simulink model "simulation_plaque"  (R2019a)
settings: Solver=ode45  StartTime=0.0  StopTime=tfin  FixedStep=0.001  RelTol=1e-09  EnableMultiTasking=on
undefined symbols (not defined in the file or in its folder): Ae, As, Be, g, Jx, LL, mP, mS, phi_1, RR, Vmax, XA, XB, XC, XD, XE, XF, YA, YB, YC, YD, YE, YF, z_re
settings Model: Creator=delafontaine  LastModifiedBy=arsp2701
settings SolverCC: AlgebraicLoopSolver=LineSearch
settings DataIOCC: LimitDataPoints=on  SaveFormat=Array  SignalLoggingSaveFormat=ModelDataLogs  ReturnWorkspaceOutputs=off
settings OptimizationCC: LifeSpan=inf
settings DebuggingCC: UnderspecifiedInitializationDetection=Classic  MergeDetectMultiDrivingBlocksExec=none  MultiTaskDSMMsg=warning  MultiTaskCondExecSysMsg=none  SFUnexpectedBacktrackingDiag=warning  SFNoUnconditionalDefaultTransitionDiag=warning  SFExecutionAtInitializationDiag=none  UnderSpecifiedDimensionMsg=warning  ArithmeticOperatorsInVariantConditions=warning
settings HardwareCC: ProdBitPerPointer=32  ProdBitPerSizeT=32  ProdBitPerPtrDiffT=32  ProdLargestAtomicFloat=None  ProdIntDivRoundTo=Undefined  ProdEndianess=Unspecified  ProdWordSize=32  ProdHWDeviceType=32-bit Generic
settings ModelReferenceCC: PropagateSignalLabelsOutOfModel=off
settings SFSimCC: SimUseLocalCustomCode=off
settings RTWCC: RTWUseLocalCustomCode=off
settings CodeAppCC: StateflowObjectComments=on
settings GRTTargetCC: TargetLangStandard=C89/C90 (ANSI)  GeneratePreprocessorConditionals=Disable all
settings ConfigComp: CovMetricSettings=dw  CovHtmlReporting=on  CovSaveCumulativeToWorkspaceVar=on  CovSaveSingleToWorkspaceVar=on  CovExternalEMLEnable=off  CovSFcnEnable=off

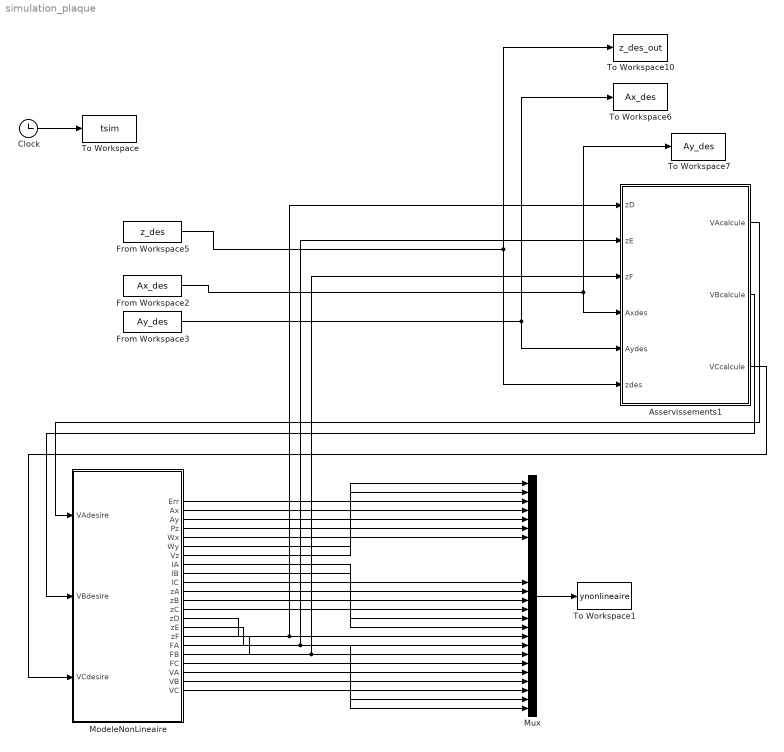
== system simulation_plaque ==
  Asservissements1 : Subsystem
      mask help: Simulink:masks:GenSFuncDesc_MD
      mask Help: eval('feval(''rtwprivate'',''rtwhelpview'',''rtw_sfcn_block'')');
  Clock : Clock
  From Workspace2 : FromWorkspace  VariableName=Ax_des  SampleTime=0  Interpolate=off  OutputAfterFinalValue=Holding final value
  From Workspace3 : FromWorkspace  VariableName=Ay_des  SampleTime=0  Interpolate=off  OutputAfterFinalValue=Holding final value
  From Workspace5 : FromWorkspace  VariableName=z_des  SampleTime=0  Interpolate=off  OutputAfterFinalValue=Holding final value
  ModeleNonLineaire : Subsystem
      mask help: Simulink:masks:GenSFuncDesc_MD
      mask Help: eval('feval(''rtwprivate'',''rtwhelpview'',''rtw_sfcn_block'')');
  Mux : Mux  Inputs=26
  To Workspace : ToWorkspace  VariableName=tsim  SampleTime=-1
  To Workspace1 : ToWorkspace  VariableName=ynonlineaire  SampleTime=-1
  To Workspace10 : ToWorkspace  VariableName=z_des_out  SampleTime=-1
  To Workspace6 : ToWorkspace  VariableName=Ax_des  SampleTime=-1
  To Workspace7 : ToWorkspace  VariableName=Ay_des  SampleTime=-1
  wires:
  Mux/1 -> To Workspace1/1
  Clock/1 -> To Workspace/1
  From Workspace5/1 -> Asservissements1/6(zdes), To Workspace10/1
  ModeleNonLineaire/2(Ax) -> Mux/2
  ModeleNonLineaire/3(Ay) -> Mux/3
  ModeleNonLineaire/4(Pz) -> Mux/4
  ModeleNonLineaire/5(Wx) -> Mux/5
  ModeleNonLineaire/6(Wy) -> Mux/6
  ModeleNonLineaire/7(Vz) -> Mux/7
  ModeleNonLineaire/8(IA) -> Mux/12
  ModeleNonLineaire/9(IB) -> Mux/13
  ModeleNonLineaire/10(IC) -> Mux/14
  From Workspace3/1 -> To Workspace6/1, Asservissements1/5(Aydes)
  From Workspace2/1 -> To Workspace7/1, Asservissements1/4(Axdes)
  ModeleNonLineaire/17(FA) -> Mux/21
  ModeleNonLineaire/18(FB) -> Mux/22
  ModeleNonLineaire/19(FC) -> Mux/23
  ModeleNonLineaire/20(VA) -> Mux/24
  ModeleNonLineaire/21(VB) -> Mux/25
  ModeleNonLineaire/22(VC) -> Mux/26
  ModeleNonLineaire/14(zD) -> Asservissements1/1(zD), Mux/18
  ModeleNonLineaire/15(zE) -> Asservissements1/2(zE), Mux/19
  ModeleNonLineaire/16(zF) -> Asservissements1/3(zF), Mux/20
  ModeleNonLineaire/11(zA) -> Mux/15
  ModeleNonLineaire/12(zB) -> Mux/16
  ModeleNonLineaire/13(zC) -> Mux/17
  Asservissements1/1(VAcalcule) -> ModeleNonLineaire/1(VAdesire)
  Asservissements1/2(VBcalcule) -> ModeleNonLineaire/2(VBdesire)
  Asservissements1/3(VCcalcule) -> ModeleNonLineaire/3(VCdesire)
  ModeleNonLineaire/1("Err ") -> Mux/1

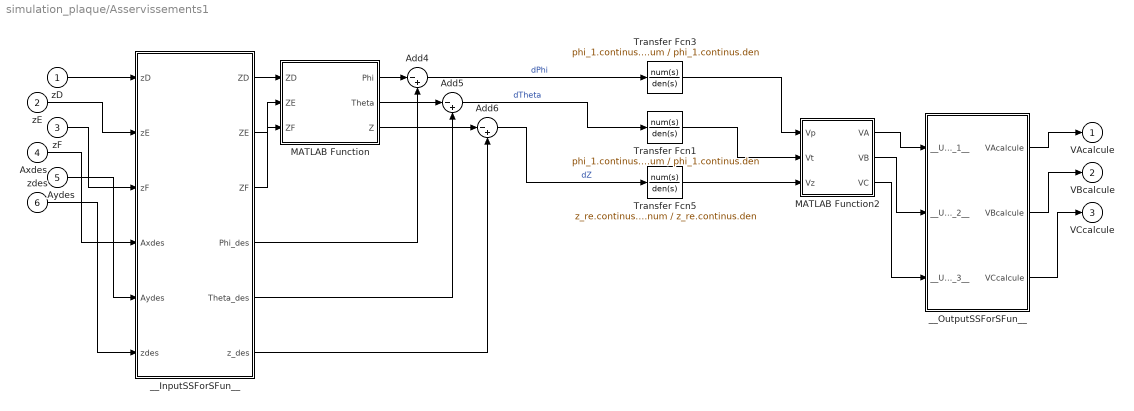
== system simulation_plaque/Asservissements1 ==
  zD : Inport
  zE : Inport  Port=2
  zF : Inport  Port=3
  Axdes : Inport  Port=4
  Aydes : Inport  Port=5
  zdes : Inport  Port=6
  Add4 : Sum  Inputs=|-+
  Add5 : Sum  Inputs=|-+
  Add6 : Sum  Inputs=|-+
  MATLAB Function : MATLAB Function  TreatAsAtomicUnit=on
  MATLAB Function2 : MATLAB Function  TreatAsAtomicUnit=on
  Transfer Fcn1 : TransferFcn  Numerator=phi_1.continus.num  Denominator=phi_1.continus.den
  Transfer Fcn3 : TransferFcn  Numerator=phi_1.continus.num  Denominator=phi_1.continus.den
  Transfer Fcn5 : TransferFcn  Numerator=z_re.continus.num  Denominator=z_re.continus.den
  __InputSSForSFun__ : Subsystem
  __OutputSSForSFun__ : Subsystem
  VAcalcule : Outport
  VBcalcule : Outport  Port=2
  VCcalcule : Outport  Port=3
  wires:
  zD/1 -> __InputSSForSFun__/1(zD)
  zE/1 -> __InputSSForSFun__/2(zE)
  zF/1 -> __InputSSForSFun__/3(zF)
  Axdes/1 -> __InputSSForSFun__/4(Axdes)
  Aydes/1 -> __InputSSForSFun__/5(Aydes)
  zdes/1 -> __InputSSForSFun__/6(zdes)
  __InputSSForSFun__/1(ZD) -> MATLAB Function/1(ZD)
  __OutputSSForSFun__/1(VAcalcule) -> VAcalcule/1
  __OutputSSForSFun__/2(VBcalcule) -> VBcalcule/1
  __OutputSSForSFun__/3(VCcalcule) -> VCcalcule/1
  MATLAB Function/1(Phi) -> Add4/1
  MATLAB Function/3(Z) -> Add6/1
  MATLAB Function2/1(VA) -> __OutputSSForSFun__/1(__UniqueInportName__1__)
  MATLAB Function2/2(VB) -> __OutputSSForSFun__/2(__UniqueInportName__2__)
  MATLAB Function2/3(VC) -> __OutputSSForSFun__/3(__UniqueInportName__3__)
  MATLAB Function/2(Theta) -> Add5/1
  Add4/1 -> Transfer Fcn3/1  "dPhi"
  Transfer Fcn3/1 -> MATLAB Function2/1(Vp)
  Transfer Fcn1/1 -> MATLAB Function2/2(Vt)
  Add5/1 -> Transfer Fcn1/1  "dTheta"
  Transfer Fcn5/1 -> MATLAB Function2/3(Vz)
  Add6/1 -> Transfer Fcn5/1  "dZ"
  __InputSSForSFun__/2(ZE) -> MATLAB Function/2(ZE)
  __InputSSForSFun__/3(ZF) -> MATLAB Function/3(ZF)
  __InputSSForSFun__/4(Phi_des) -> Add4/2
  __InputSSForSFun__/5(Theta_des) -> Add5/2
  __InputSSForSFun__/6(z_des) -> Add6/2

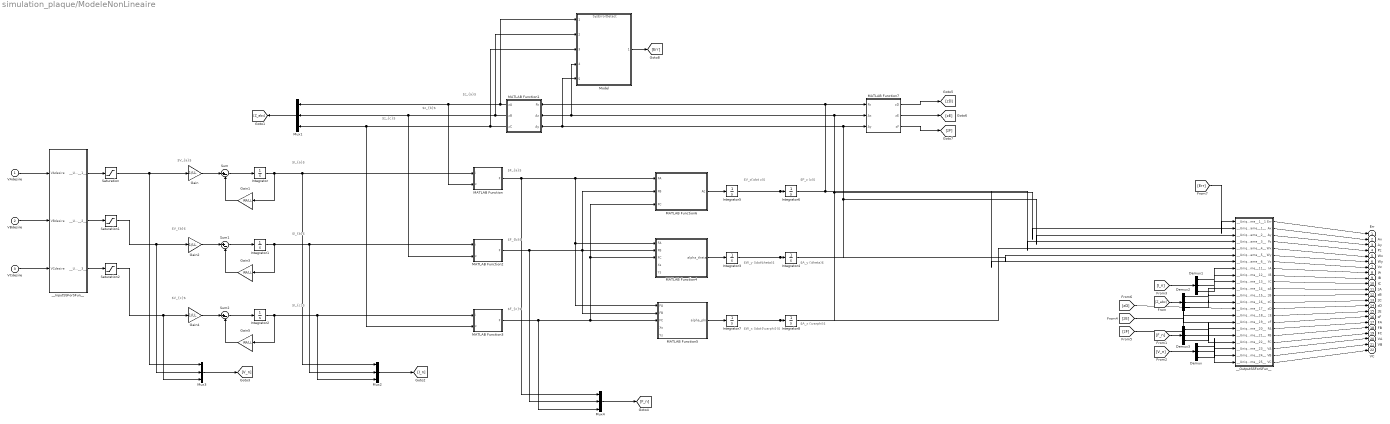
== system simulation_plaque/ModeleNonLineaire ==
  note: $z_{c}$
  note: $I_{a}$
  note: $I_{c}$
  note: $z_{b}$
  note: $F_{a}$
  note: $V_{b}$
  note: $F_{b}$
  note: $F_{c}$
  note: $V_{c}$
  note: $V_z(\dot z)$
  note: $z_{a}$
  note: $I_{b}$
  note: $V_{a}$
  note: $A_y (\theta)$
  note: $A_x (\varphi)$
  note: $W_x (\dot{\varphi})$
  note: $W_y (\dot\theta)$
  note: $P_z (z)$
  VAdesire : Inport
  VBdesire : Inport  Port=2
  VCdesire : Inport  Port=3
  Demux{,1..3} (4 alike) : Demux  Outputs=3
  Gain : Gain  Gain=1/LL
  Gain1 : Gain  Gain=RR/LL
  Gain2 : Gain  Gain=1/LL
  Gain3 : Gain  Gain=RR/LL
  Gain4 : Gain  Gain=1/LL
  Gain5 : Gain  Gain=RR/LL
  Integrator : Integrator  InitialCondition=-0.4961
  Integrator1 : Integrator  InitialCondition=-0.4961
  Integrator2 : Integrator  InitialCondition=-0.4961
  Integrator{3..5,7..8} (5 alike) : Integrator
  Integrator6 : Integrator  InitialCondition=0.015
  MATLAB Function : MATLAB Function  TreatAsAtomicUnit=on
  MATLAB Function1 : MATLAB Function  TreatAsAtomicUnit=on
  MATLAB Function2 : MATLAB Function  TreatAsAtomicUnit=on
  MATLAB Function3 : MATLAB Function  TreatAsAtomicUnit=on
  MATLAB Function4 : MATLAB Function  TreatAsAtomicUnit=on
  MATLAB Function5 : MATLAB Function  TreatAsAtomicUnit=on
  MATLAB Function6 : MATLAB Function  TreatAsAtomicUnit=on
  MATLAB Function7 : MATLAB Function  TreatAsAtomicUnit=on
  Model : ModelReference  ModelNameDialog=SysErrorDetect.slx  SimulationMode=Normal  ModelReferenceVersion=1.36
  Mux{1..4} (4 alike) : Mux  Inputs=3
  Saturation : Saturate  UpperLimit=Vmax  LowerLimit=-Vmax
  Saturation1 : Saturate  UpperLimit=Vmax  LowerLimit=-Vmax
  Saturation2 : Saturate  UpperLimit=Vmax  LowerLimit=-Vmax
  Sum : Sum  Inputs=|+-
  Sum1 : Sum  Inputs=|+-
  Sum2 : Sum  Inputs=|+-
  __InputSSForSFun__ : Subsystem
  __OutputSSForSFun__ : Subsystem
  "Err " : Outport
  Ax : Outport  Port=2
  Ay : Outport  Port=3
  Pz : Outport  Port=4
  Wx : Outport  Port=5
  Wy : Outport  Port=6
  Vz : Outport  Port=7
  IA : Outport  Port=8
  IB : Outport  Port=9
  IC : Outport  Port=10
  zA : Outport  Port=11
  zB : Outport  Port=12
  zC : Outport  Port=13
  zD : Outport  Port=14
  zE : Outport  Port=15
  zF : Outport  Port=16
  FA : Outport  Port=17
  FB : Outport  Port=18
  FC : Outport  Port=19
  VA : Outport  Port=20
  VB : Outport  Port=21
  VC : Outport  Port=22
  wires:
  VAdesire/1 -> __InputSSForSFun__/1(VAdesire)
  VBdesire/1 -> __InputSSForSFun__/2(VBdesire)
  VCdesire/1 -> __InputSSForSFun__/3(VCdesire)
  __InputSSForSFun__/1(__UniqueOutportName__1__) -> Saturation/1
  __InputSSForSFun__/2(__UniqueOutportName__2__) -> Saturation1/1
  __InputSSForSFun__/3(__UniqueOutportName__3__) -> Saturation2/1
  __OutputSSForSFun__/2(Ax) -> Ax/1
  __OutputSSForSFun__/3(Ay) -> Ay/1
  __OutputSSForSFun__/4(Pz) -> Pz/1
  __OutputSSForSFun__/5(Wx) -> Wx/1
  __OutputSSForSFun__/6(Wy) -> Wy/1
  __OutputSSForSFun__/7(Vz) -> Vz/1
  __OutputSSForSFun__/8(IA) -> IA/1
  __OutputSSForSFun__/9(IB) -> IB/1
  __OutputSSForSFun__/10(IC) -> IC/1
  __OutputSSForSFun__/11(zA) -> zA/1
  __OutputSSForSFun__/12(zB) -> zB/1
  __OutputSSForSFun__/13(zC) -> zC/1
  __OutputSSForSFun__/14(zD) -> zD/1
  __OutputSSForSFun__/15(zE) -> zE/1
  __OutputSSForSFun__/16(zF) -> zF/1
  __OutputSSForSFun__/17(FA) -> FA/1
  __OutputSSForSFun__/18(FB) -> FB/1
  __OutputSSForSFun__/19(FC) -> FC/1
  __OutputSSForSFun__/20(VA) -> VA/1
  __OutputSSForSFun__/21(VB) -> VB/1
  __OutputSSForSFun__/22(VC) -> VC/1
  Sum2/1 -> Integrator2/1
  Integrator/1 -> MATLAB Function/1(i), Mux2/1, Gain1/1
  Integrator8/1 -> __OutputSSForSFun__/2(__UniqueInportName__1__), Model/4, MATLAB Function1/2(Ax), MATLAB Function7/2(Ax)
  Integrator1/1 -> MATLAB Function2/1(i), Mux2/2, Gain3/1
  MATLAB Function1/3(zC) -> Model/3, MATLAB Function3/2(z), Mux1/3
  MATLAB Function/1(F) -> Mux4/1, MATLAB Function6/1(FA), MATLAB Function4/1(FA), MATLAB Function5/1(FA)
  Sum1/1 -> Integrator1/1
  MATLAB Function5/1(alpha_phi) -> Integrator7/1
  MATLAB Function6/1(Az) -> Integrator5/1
  Sum/1 -> Integrator/1
  Gain3/1 -> Sum1/2
  Integrator2/1 -> Gain5/1, MATLAB Function3/1(i), Mux2/3
  Integrator7/1 -> Integrator8/1, __OutputSSForSFun__/5(__UniqueInportName__4__)
  Gain5/1 -> Sum2/2
  MATLAB Function1/1(zA) -> Model/1, MATLAB Function/2(z), Mux1/1
  Integrator6/1 -> MATLAB Function1/1(Pz), MATLAB Function7/1(Pz), __OutputSSForSFun__/4(__UniqueInportName__3__)
  Integrator3/1 -> __OutputSSForSFun__/6(__UniqueInportName__5__), Integrator4/1
  Gain2/1 -> Sum1/1
  Integrator4/1 -> Model/5, MATLAB Function1/3(Ay), MATLAB Function7/3(Ay), __OutputSSForSFun__/3(__UniqueInportName__2__)
  MATLAB Function4/1(alpha_theta) -> Integrator3/1
  MATLAB Function3/1(F) -> Mux4/3, MATLAB Function5/3(FC), MATLAB Function4/3(FC), MATLAB Function6/3(FC)
  Gain/1 -> Sum/1
  Gain4/1 -> Sum2/1
  MATLAB Function2/1(F) -> Mux4/2, MATLAB Function4/2(FB), MATLAB Function6/2(FB), MATLAB Function5/2(FB)
  Gain1/1 -> Sum/2
  MATLAB Function1/2(zB) -> Model/2, MATLAB Function2/2(z), Mux1/2
  Integrator5/1 -> Integrator6/1, __OutputSSForSFun__/7(__UniqueInportName__6__)
  Mux1/1 -> [Z_abc]
  Mux2/1 -> [I_n]
  Mux3/1 -> [V_n]
  Demux/1 -> __OutputSSForSFun__/20(__UniqueInportName__23__)
  Demux/2 -> __OutputSSForSFun__/21(__UniqueInportName__24__)
  Demux/3 -> __OutputSSForSFun__/22(__UniqueInportName__25__)
  [V_n] -> Demux/1
  Demux1/1 -> __OutputSSForSFun__/8(__UniqueInportName__11__)
  Demux1/2 -> __OutputSSForSFun__/9(__UniqueInportName__12__)
  Demux1/3 -> __OutputSSForSFun__/10(__UniqueInportName__13__)
  [I_n] -> Demux1/1
  Demux2/1 -> __OutputSSForSFun__/11(__UniqueInportName__14__)
  Demux2/2 -> __OutputSSForSFun__/12(__UniqueInportName__15__)
  Demux2/3 -> __OutputSSForSFun__/13(__UniqueInportName__16__)
  [Z_abc] -> Demux2/1
  Mux4/1 -> [F_n]
  [F_n] -> Demux3/1
  Demux3/3 -> __OutputSSForSFun__/19(__UniqueInportName__22__)
  Demux3/2 -> __OutputSSForSFun__/18(__UniqueInportName__21__)
  Demux3/1 -> __OutputSSForSFun__/17(__UniqueInportName__20__)
  [zD] -> __OutputSSForSFun__/14(__UniqueInportName__17__)
  [zE] -> __OutputSSForSFun__/15(__UniqueInportName__18__)
  [zF] -> __OutputSSForSFun__/16(__UniqueInportName__19__)
  MATLAB Function7/1(zD) -> [zD]
  MATLAB Function7/2(zE) -> [zE]
  MATLAB Function7/3(zF) -> [zF]
  Saturation/1 -> Gain/1, Mux3/1
  Saturation1/1 -> Mux3/2, Gain2/1
  Saturation2/1 -> Mux3/3, Gain4/1
  [Err] -> __OutputSSForSFun__/1(__UniqueInportName__1__1)
  Model/1 -> [Err]
  __OutputSSForSFun__/1(Err) -> "Err "/1

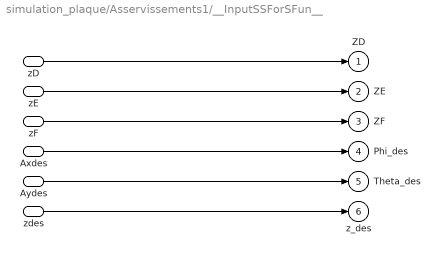
== system simulation_plaque/Asservissements1/__InputSSForSFun__ ==
  zD : Inport
  zE : Inport  Port=2
  zF : Inport  Port=3
  Axdes : Inport  Port=4
  Aydes : Inport  Port=5
  zdes : Inport  Port=6
  ZD : Outport
  ZE : Outport  Port=2
  ZF : Outport  Port=3
  Phi_des : Outport  Port=4
  Theta_des : Outport  Port=5
  z_des : Outport  Port=6
  wires:
  zD/1 -> ZD/1
  zE/1 -> ZE/1
  zF/1 -> ZF/1
  Axdes/1 -> Phi_des/1
  Aydes/1 -> Theta_des/1
  zdes/1 -> z_des/1

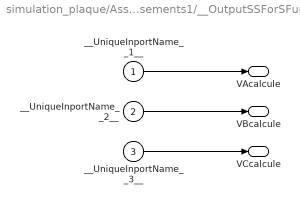
== system simulation_plaque/Asservissements1/__OutputSSForSFun__ ==
  __UniqueInportName__1__ : Inport
  __UniqueInportName__2__ : Inport  Port=2
  __UniqueInportName__3__ : Inport  Port=3
  VAcalcule : Outport
  VBcalcule : Outport  Port=2
  VCcalcule : Outport  Port=3
  wires:
  __UniqueInportName__1__/1 -> VAcalcule/1
  __UniqueInportName__2__/1 -> VBcalcule/1
  __UniqueInportName__3__/1 -> VCcalcule/1

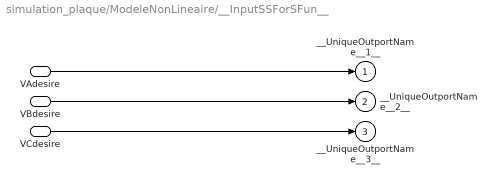
== system simulation_plaque/ModeleNonLineaire/__InputSSForSFun__ ==
  VAdesire : Inport
  VBdesire : Inport  Port=2
  VCdesire : Inport  Port=3
  __UniqueOutportName__1__ : Outport
  __UniqueOutportName__2__ : Outport  Port=2
  __UniqueOutportName__3__ : Outport  Port=3
  wires:
  VAdesire/1 -> __UniqueOutportName__1__/1
  VBdesire/1 -> __UniqueOutportName__2__/1
  VCdesire/1 -> __UniqueOutportName__3__/1

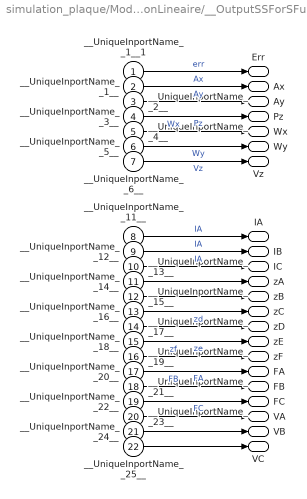
== system simulation_plaque/ModeleNonLineaire/__OutputSSForSFun__ ==
  __UniqueInportName__1__1 : Inport
  __UniqueInportName__1__ : Inport  Port=2
  __UniqueInportName__2__ : Inport  Port=3
  __UniqueInportName__3__ : Inport  Port=4
  __UniqueInportName__4__ : Inport  Port=5
  __UniqueInportName__5__ : Inport  Port=6
  __UniqueInportName__6__ : Inport  Port=7
  __UniqueInportName__11__ : Inport  Port=8
  __UniqueInportName__12__ : Inport  Port=9
  __UniqueInportName__13__ : Inport  Port=10
  __UniqueInportName__14__ : Inport  Port=11
  __UniqueInportName__15__ : Inport  Port=12
  __UniqueInportName__16__ : Inport  Port=13
  __UniqueInportName__17__ : Inport  Port=14
  __UniqueInportName__18__ : Inport  Port=15
  __UniqueInportName__19__ : Inport  Port=16
  __UniqueInportName__20__ : Inport  Port=17
  __UniqueInportName__21__ : Inport  Port=18
  __UniqueInportName__22__ : Inport  Port=19
  __UniqueInportName__23__ : Inport  Port=20
  __UniqueInportName__24__ : Inport  Port=21
  __UniqueInportName__25__ : Inport  Port=22
  Err : Outport
  Ax : Outport  Port=2
  Ay : Outport  Port=3
  Pz : Outport  Port=4
  Wx : Outport  Port=5
  Wy : Outport  Port=6
  Vz : Outport  Port=7
  IA : Outport  Port=8
  IB : Outport  Port=9
  IC : Outport  Port=10
  zA : Outport  Port=11
  zB : Outport  Port=12
  zC : Outport  Port=13
  zD : Outport  Port=14
  zE : Outport  Port=15
  zF : Outport  Port=16
  FA : Outport  Port=17
  FB : Outport  Port=18
  FC : Outport  Port=19
  VA : Outport  Port=20
  VB : Outport  Port=21
  VC : Outport  Port=22
  wires:
  __UniqueInportName__1__/1 -> Ax/1  "Ax"
  __UniqueInportName__2__/1 -> Ay/1  "Ay"
  __UniqueInportName__3__/1 -> Pz/1  "Pz"
  __UniqueInportName__4__/1 -> Wx/1  "Wx"
  __UniqueInportName__5__/1 -> Wy/1  "Wy"
  __UniqueInportName__6__/1 -> Vz/1  "Vz"
  __UniqueInportName__11__/1 -> IA/1  "IA"
  __UniqueInportName__12__/1 -> IB/1  "IA"
  __UniqueInportName__13__/1 -> IC/1  "IA"
  __UniqueInportName__14__/1 -> zA/1
  __UniqueInportName__15__/1 -> zB/1
  __UniqueInportName__16__/1 -> zC/1
  __UniqueInportName__17__/1 -> zD/1  "zd"
  __UniqueInportName__18__/1 -> zE/1  "ze"
  __UniqueInportName__19__/1 -> zF/1  "zf"
  __UniqueInportName__20__/1 -> FA/1  "FA"
  __UniqueInportName__21__/1 -> FB/1  "FB"
  __UniqueInportName__22__/1 -> FC/1  "FC"
  __UniqueInportName__23__/1 -> VA/1
  __UniqueInportName__24__/1 -> VB/1
  __UniqueInportName__25__/1 -> VC/1
  __UniqueInportName__1__1/1 -> Err/1  "err"

== matlab function simulation_plaque/ModeleNonLineaire/MATLAB Function1 ==
  data: Pz input; Ax input; zA output double size=1; Ay input; zB output double size=1; zC output double size=1; XA parameter size=1; XB parameter size=1; XC parameter size=1; YA parameter size=1; YB parameter size=1; YC parameter size=1
function [zA,zB,zC] = fcn(Pz, Ax , Ay, XA, XB, XC, YA, YB, YC)

    zA = Pz- XA*Ay + YA*Ax;
    
    zB = Pz- XB*Ay + YB*Ax;
    
    zC = Pz- XC*Ay + YC*Ax;

== matlab function simulation_plaque/ModeleNonLineaire/MATLAB Function ==
  data: i input size=1; F output double size=1; z input size=1; Ae parameter size=4; As parameter size=4; Be parameter size=1
function F = fcn(i , z, Ae, As, Be)

    FSK = -1/(As(1) + As(2)*z + As(3)*z^2 +As(4)*z^3);
    
    FEK = ((i^2 + Be*abs(i))*sign(i))/(Ae(1) + Ae(2)*z + Ae(3)*z^2 + Ae(4)*z^3);

    F = FEK + FSK;

== matlab function simulation_plaque/ModeleNonLineaire/MATLAB Function2 ==
  data: i input size=1; F output double size=1; z input size=1; Ae parameter size=4; As parameter size=4; Be parameter size=1
function F = fcn(i , z, Ae, As, Be)

    FSK = -1/(As(1) + As(2)*z + As(3)*z^2 +As(4)*z^3);
    
    FEK = ((i^2 + Be*abs(i))*sign(i))/(Ae(1) + Ae(2)*z + Ae(3)*z^2 + Ae(4)*z^3);

    F = FEK + FSK;

== matlab function simulation_plaque/ModeleNonLineaire/MATLAB Function3 ==
  data: i input size=1; F output double size=1; z input size=1; Ae parameter size=4; As parameter size=4; Be parameter size=1
function F = fcn(i , z, Ae, As, Be)

    FSK = -1/(As(1) + As(2)*z + As(3)*z^2 +As(4)*z^3);
    
    FEK = ((i^2 + Be*abs(i))*sign(i))/(Ae(1) + Ae(2)*z + Ae(3)*z^2 + Ae(4)*z^3);

    F = FEK + FSK;

== matlab function simulation_plaque/ModeleNonLineaire/MATLAB Function4 ==
  data: FA input; alpha_theta output double size=1; FB input; FC input; Xs input; Ys input; Jx parameter size=1; mS parameter size=1; mP parameter size=1; g parameter size=1; XA parameter size=1; XB parameter size=1; XC parameter size=1
function alpha_theta = fcn(FA , FB , FC, Xs , Ys, Jx, mS, mP, g, XA, XB, XC)
    %Ay
    alpha_theta = (1/Jx)*(-FA*XA - FB*XB - FC*XC - Xs*mS*g);

== matlab function simulation_plaque/ModeleNonLineaire/MATLAB Function5 ==
  data: FA input; alpha_phi output double size=1; FB input; FC input; Xs input; Ys input; mS parameter size=1; mP parameter size=1; g parameter size=1; Jx parameter size=1; YA parameter size=1; YB parameter size=1; YC parameter size=1
function alpha_phi = fcn(FA , FB , FC, Xs , Ys, mS, mP, g, Jx, YA, YB, YC)

    alpha_phi = (1/Jx)*(FA*YA + FB*YB + FC*YC + mS*g*Ys);

== matlab function simulation_plaque/ModeleNonLineaire/MATLAB Function6 ==
  data: FA input; Az output double size=1; FB input; FC input; mS parameter size=1; mP parameter size=1; g parameter size=1
function Az = fcn(FA , FB , FC, mS, mP, g)

    Az = (FA + FB + FC + mS*g + mP*g)/mP;

== matlab function simulation_plaque/ModeleNonLineaire/MATLAB Function7 ==
  data: Pz input size=1; Ax input size=1; zD output double size=1; Ay input size=1; zE output double size=1; zF output double size=1; XD parameter size=1; YD parameter size=1; XE parameter size=1; YE parameter size=1; XF parameter size=1; YF parameter size=1
function [zD,zE,zF] = fcn(Pz , Ax , Ay, XD, YD, XE, YE, XF, YF)

    zD = Pz- XD*Ay + YD*Ax;
    
    zE = Pz- XE*Ay + YE*Ax;
    
    zF = Pz- XF*Ay + YF*Ax;

== matlab function simulation_plaque/Asservissements1/MATLAB Function ==
  data: ZD input; ZE input; ZF input; Phi output double; Theta output double; Z output double; YD parameter; YE parameter; YF parameter; XD parameter; XE parameter; XF parameter
function [Phi,Theta,Z] = fcn(ZD,ZE,ZF, YD, YE, YF, XD, XE, XF)
MOY = (ZF+ZD)/2;
Phi = (ZD-ZF)/(YD+abs(YF));
Theta = (ZE-MOY)/(XD+abs(XE));
Z = (ZD+ZE+ZF)/3;

== matlab function simulation_plaque/Asservissements1/MATLAB Function2 ==
  data: VA output; VB output; Vp input; Vt input; Vz input; VC output; YA parameter size=1; YB parameter size=1; YC parameter size=1; XA parameter size=1; XB parameter size=1; XC parameter size=1
function [VA,VB,VC] = fcn(Vp, Vt, Vz, YA, YB, YC, XA, XB, XC)
% V=[0;0;0];
U = [YA YB  YC;
    -XA -XB -XC;
    1   1   1];

Uinv = inv(U);
V = Uinv*[Vp,Vt,Vz]';

VA = V(1);
VB = V(2);
VC = V(3);
